simulink model "ws3_step_interactive_2019b"  (R2020b)
settings: Solver=FixedStepAuto  StartTime=0.0  StopTime=inf  FixedStep=1e-3
libraries: simulink x3
settings Model: Creator=jamess  LastModifiedBy=leoyi
settings DataIOCC: ReturnWorkspaceOutputs=off
settings OptimizationCC: LifeSpan=inf
settings DebuggingCC: ArithmeticOperatorsInVariantConditions=warning
settings SFSimCC: SimUseLocalCustomCode=off  CustomCodeUndefinedFunction=UseInterfaceOnly
settings RTWCC: RTWUseLocalCustomCode=off
settings CodeAppCC: StateflowObjectComments=on

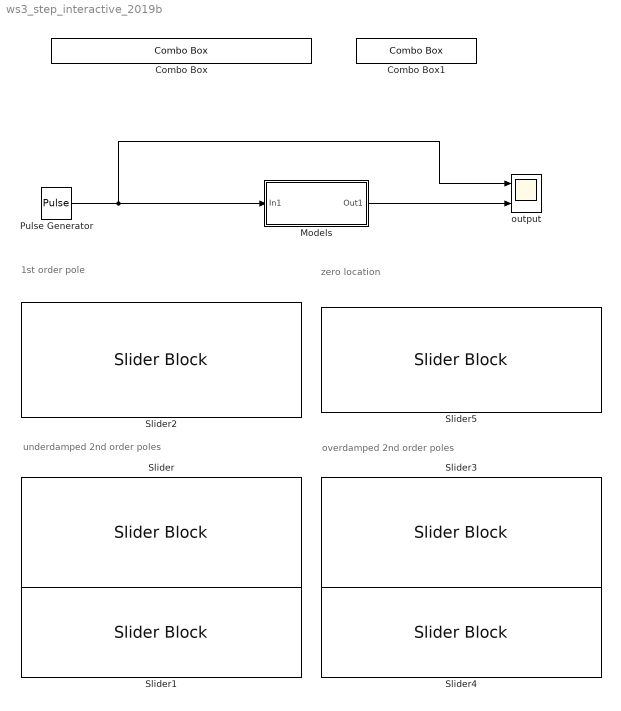
== system ws3_step_interactive_2019b ==
  note: zero location
  note: overdamped 2nd order poles
  note: underdamped 2nd order poles
  note: 1st order pole
  Combo Box : ComboBox  LabelPosition=Hide  SelectedLabel=first order
      settings: Values={{'first order', 'underdamped second order', 'overdamped second order'}, [0 1 2]}
  Combo Box1 : ComboBox  LabelPosition=Hide  SelectedLabel=no zero
      settings: Values={{'no zero', 'zero'}, [0 1]}
  Models : Subsystem
  Pulse Generator : DiscretePulseGenerator  PulseType=Time based  Period=10  PulseWidth=50
  Slider{,2..4} (4 alike) : SliderBlock  ScaleMin=-10  ScaleMax=-1  TickInterval=1
  Slider1 : SliderBlock  ScaleMax=10  TickInterval=1
  Slider5 : SliderBlock  ScaleMin=-10  ScaleMax=10  TickInterval=2
  output : Scope  NumInputPorts=2
  wires:
  Pulse Generator/1 -> output/1, Models/1(In1)
  Models/1(Out1) -> output/2

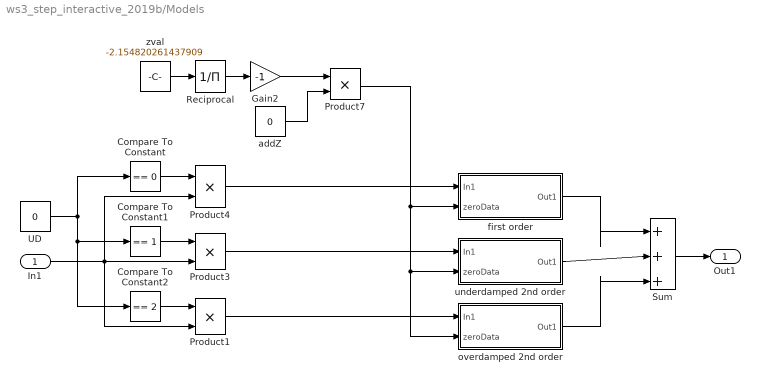
== system ws3_step_interactive_2019b/Models ==
  In1 : Inport
  Compare To Constant : simulink/Logic and Bit Operations/Compare To Constant  relop===  const=0  OutDataTypeStr=uint8
  Compare To Constant1 : simulink/Logic and Bit Operations/Compare To Constant  relop===  const=1  OutDataTypeStr=uint8
  Compare To Constant2 : simulink/Logic and Bit Operations/Compare To Constant  relop===  const=2  OutDataTypeStr=uint8
  Gain2 : Gain  Gain=-1
  Product{1,3..4,7} (4 alike) : Product
  Reciprocal : Product  Inputs=/
  Sum : Sum  Inputs=|+++
  UD : Constant  Value=0
  addZ : Constant  Value=0
  first order : Subsystem
  overdamped 2nd order : Subsystem
  underdamped 2nd order : Subsystem
  zval : Constant  Value=-2.154820261437909
  Out1 : Outport
  wires:
  In1/1 -> Product1/2, Product3/2, Product4/2
  Product1/1 -> overdamped 2nd order/1(In1)
  Product3/1 -> underdamped 2nd order/1(In1)
  Product4/1 -> first order/1(In1)
  Compare To Constant/1 -> Product4/1
  UD/1 -> Compare To Constant2/1, Compare To Constant1/1, Compare To Constant/1
  Compare To Constant1/1 -> Product3/1
  Compare To Constant2/1 -> Product1/1
  underdamped 2nd order/1(Out1) -> Sum/2
  first order/1(Out1) -> Sum/1
  overdamped 2nd order/1(Out1) -> Sum/3
  Sum/1 -> Out1/1
  Gain2/1 -> Product7/1
  Reciprocal/1 -> Gain2/1
  zval/1 -> Reciprocal/1
  addZ/1 -> Product7/2
  Product7/1 -> first order/2(zeroData), overdamped 2nd order/2(zeroData), underdamped 2nd order/2(zeroData)

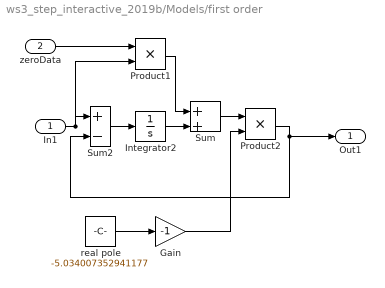
== system ws3_step_interactive_2019b/Models/first order ==
  In1 : Inport
  zeroData : Inport  Port=2
  Gain : Gain  Gain=-1
  Integrator2 : Integrator
  Product1 : Product
  Product2 : Product
  Sum : Sum  Inputs=|++
  Sum2 : Sum  Inputs=|+-
  real pole : Constant  Value=-5.034007352941177
  Out1 : Outport
  wires:
  Product2/1 -> Out1/1, Sum2/2
  Sum2/1 -> Integrator2/1
  In1/1 -> Product1/2, Sum2/1
  real pole/1 -> Gain/1
  Gain/1 -> Product2/2
  zeroData/1 -> Product1/1
  Integrator2/1 -> Sum/2
  Sum/1 -> Product2/1
  Product1/1 -> Sum/1

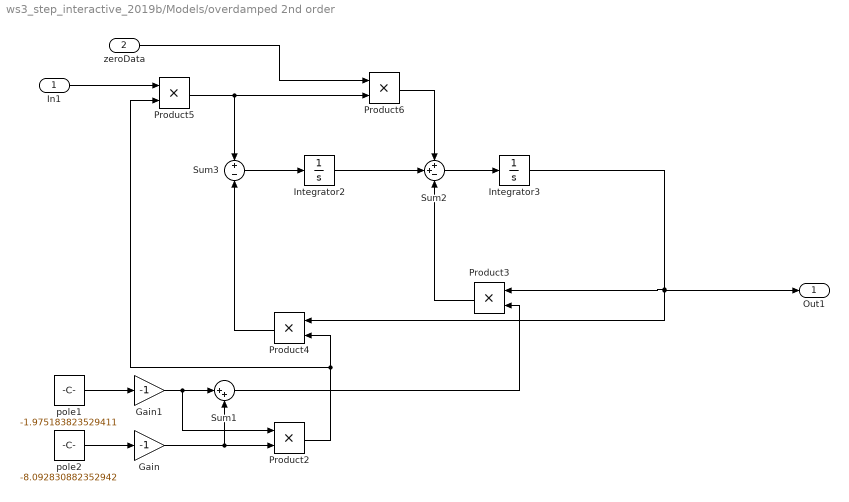
== system ws3_step_interactive_2019b/Models/overdamped 2nd order ==
  In1 : Inport
  zeroData : Inport  Port=2
  Gain : Gain  Gain=-1
  Gain1 : Gain  Gain=-1
  Integrator2 : Integrator
  Integrator3 : Integrator
  Product{2..6} (5 alike) : Product
  Sum1 : Sum  Inputs=|++
  Sum2 : Sum  Inputs=++-
  Sum3 : Sum  Inputs=+|-
  pole1 : Constant  Value=-1.975183823529411
  pole2 : Constant  Value=-8.092830882352942
  Out1 : Outport
  wires:
  pole2/1 -> Gain/1
  Gain/1 -> Sum1/2, Product2/2
  pole1/1 -> Gain1/1
  Gain1/1 -> Product2/1, Sum1/1
  Sum2/1 -> Integrator3/1
  Integrator2/1 -> Sum2/2
  Integrator3/1 -> Product4/1, Out1/1, Product3/1
  Sum1/1 -> Product3/2
  Product3/1 -> Sum2/3
  Sum3/1 -> Integrator2/1
  Product2/1 -> Product5/2, Product4/2
  Product4/1 -> Sum3/2
  In1/1 -> Product5/1
  Product5/1 -> Sum3/1, Product6/2
  Product6/1 -> Sum2/1
  zeroData/1 -> Product6/1

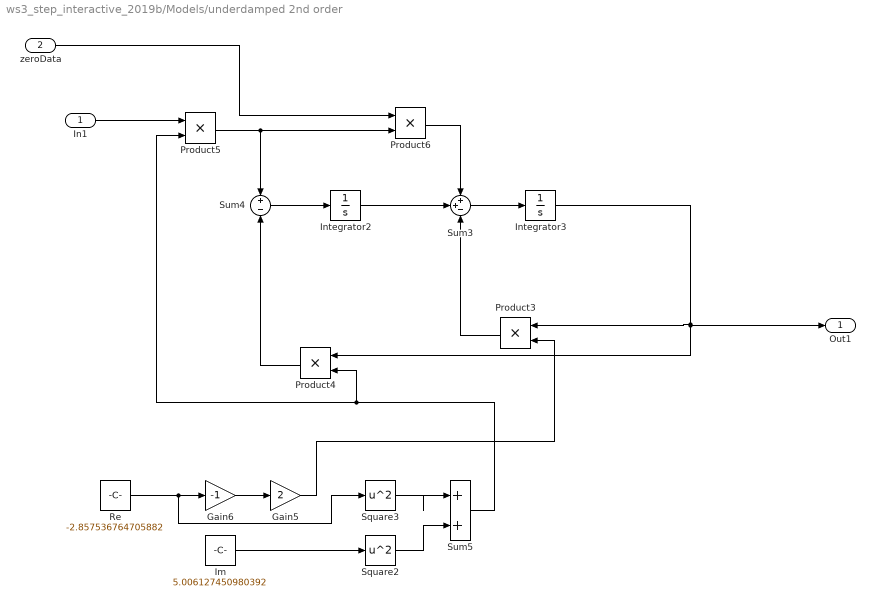
== system ws3_step_interactive_2019b/Models/underdamped 2nd order ==
  In1 : Inport
  zeroData : Inport  Port=2
  Gain5 : Gain  Gain=2
  Gain6 : Gain  Gain=-1
  Im : Constant  Value=5.006127450980392
  Integrator2 : Integrator
  Integrator3 : Integrator
  Product{3..6} (4 alike) : Product
  Re : Constant  Value=-2.857536764705882
  Square2 : Math  Operator=square  SaturateOnIntegerOverflow=on
  Square3 : Math  Operator=square  SaturateOnIntegerOverflow=on
  Sum3 : Sum  Inputs=++-
  Sum4 : Sum  Inputs=+|-
  Sum5 : Sum  Inputs=|++
  Out1 : Outport
  wires:
  zeroData/1 -> Product6/1
  Sum3/1 -> Integrator3/1
  Product5/1 -> Sum4/1, Product6/2
  Integrator2/1 -> Sum3/2
  Product4/1 -> Sum4/2
  Product3/1 -> Sum3/3
  Sum5/1 -> Product5/2, Product4/2
  Integrator3/1 -> Out1/1, Product4/1, Product3/1
  Product6/1 -> Sum3/1
  Sum4/1 -> Integrator2/1
  In1/1 -> Product5/1
  Square2/1 -> Sum5/2
  Re/1 -> Square3/1, Gain6/1
  Gain6/1 -> Gain5/1
  Square3/1 -> Sum5/1
  Gain5/1 -> Product3/2
  Im/1 -> Square2/1
